simulink model "corBO"  (R2016b)
settings: Solver=VariableStepAuto  StartTime=0.0  StopTime=10.0  RelTol=1e-3
undefined symbols (not defined in the file or in its folder): f, Ki, Kred, meq, rpignon
settings Model: Creator=canar  LastModifiedBy=canar

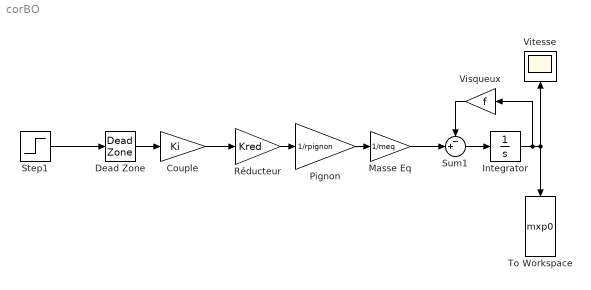
== system corBO ==
  Couple : Gain  Gain=Ki
  Dead Zone : DeadZone  LowerValue=-0.05  UpperValue=0.05  SaturateOnIntegerOverflow=on
  Integrator : Integrator
  Masse Eq : Gain  Gain=1/meq
  Pignon : Gain  Gain=1/rpignon
  Réducteur : Gain  Gain=Kred
  Step1 : Step  Time=0.1  After=0.2  SampleTime=0
  Sum1 : Sum  Inputs=-+|
  To Workspace : ToWorkspace  VariableName=mxp0  SaveFormat=Timeseries  SampleTime=-1
  Visqueux : Gain  Gain=f
  Vitesse : Scope
  wires:
  Pignon/1 -> Masse Eq/1
  Integrator/1 -> Visqueux/1, To Workspace/1, Vitesse/1
  Sum1/1 -> Integrator/1
  Visqueux/1 -> Sum1/1
  Masse Eq/1 -> Sum1/2
  Réducteur/1 -> Pignon/1
  Step1/1 -> Dead Zone/1
  Couple/1 -> Réducteur/1
  Dead Zone/1 -> Couple/1
